simulink model "Golf_Nonlin_Modale"  (R2019a)
settings: Solver=VariableStepAuto  StartTime=0.0  StopTime=300  RelTol=1e-3
values from neighbouring files (symbols this model uses):
  A6 = Acm(iVa:end, iVa:end)    [mainProjetCADV_2a.m]
  alphaTrim = trimVal(2)    [mainProjetCADV_2a.m]
  B6 = Bcm(iVa:end)    [mainProjetCADV_2a.m]
  Cobs = [C6(1,:); C6(3,:); C6(4,:)]    [mainProjetCADV_2a.m]
  Cpf = tf(q(end), minFTBF.num{1})    [mainProjetCADV_2a.m]
  dPHRTrim = trimVal(1)    [mainProjetCADV_2a.m]
  dthrIdle = 0.1    [mainProjetCADV_2a.m]
  H = -inv(C6_pour_h*inv(A6-B6*K_x)*B6)    [mainProjetCADV_2a.m]
  K_i = K_aug(end)    [mainProjetCADV_2a.m]
  K_x = K_aug(1:end-1)    [mainProjetCADV_2a.m]
  km = trim.kmass(choix)    [utGetTrimPoint.m]
  KTS2MS = 1852 / 3600    (= 0.514444444444)    [mainProjetCADV_2a.m]    (also in utAcDynamicsFunction.m)
  L6 = L6t'    [mainProjetCADV_2a.m]
  ms = trim.mStat(choix)    [utGetTrimPoint.m]
  RAD2DEG = 180/pi    (= 57.2957795131)    [mainProjetCADV_2a.m]    (also in utAcDynamicsFunction.m)
  thetaTrim = trimVal(3)    [mainProjetCADV_2a.m]
  uTrim = zeros(TOTAL_CMD, 1)    [mainProjetCADV_2a.m]
  VaTrim = utEas2Tas(Eas_KTS*KTS2MS, hTrimFL*FL2M)    [mainProjetCADV_2a.m]
  xTrim = zeros(TOTAL_SV, 1)    [mainProjetCADV_2a.m]
undefined symbols (not defined in the file or in its folder): aircraftChosen, Eas_KTS, Kd, Ki, Kp
settings Model: Creator=bourdiul  LastModifiedBy=ulyss

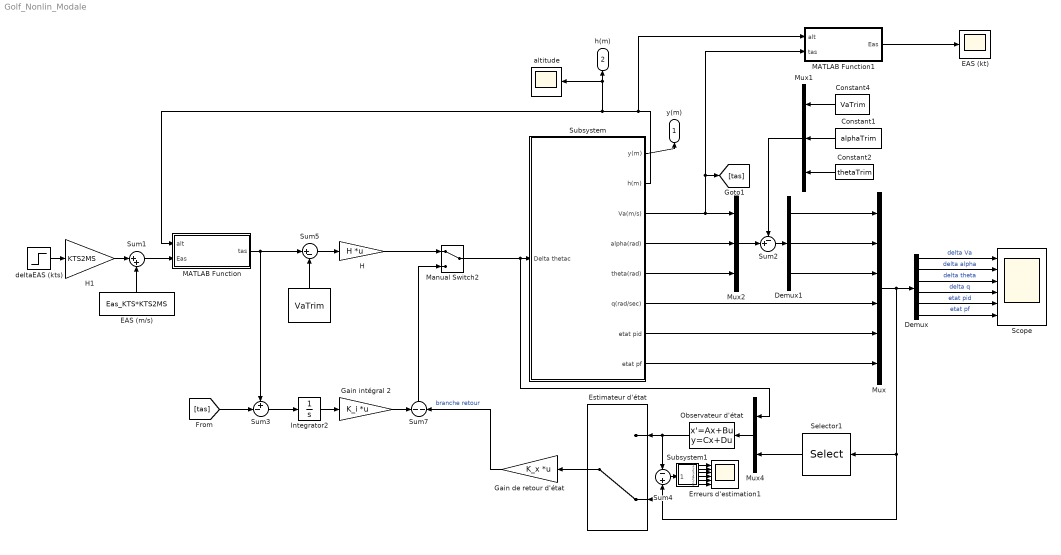
== system Golf_Nonlin_Modale ==
  " " : Constant  Value=VaTrim
  Constant1 : Constant  Value=alphaTrim
  Constant2 : Constant  Value=thetaTrim
  Constant4 : Constant  Value=VaTrim
  Demux : Demux  Outputs=6
  Demux1 : Demux  Outputs=3
  EAS (kt) : Scope
  EAS (m/s) : Constant  Value=Eas_KTS*KTS2MS
  Erreurs d'estimation1 : Scope  NumInputPorts=6
  Estimateur d'état : ManualSwitch  CurrentSetting=0
  Gain de retour d'état : Gain  Gain=K_x  Multiplication=Matrix(K*u) (u vector)
  Gain intégral 2 : Gain  Gain=K_i  Multiplication=Matrix(K*u) (u vector)
  H : Gain  Gain=H  Multiplication=Matrix(K*u) (u vector)
  H1 : Gain  Gain=KTS2MS
  Integrator2 : Integrator
  MATLAB Function : MATLAB Function  TreatAsAtomicUnit=on
  MATLAB Function1 : MATLAB Function  TreatAsAtomicUnit=on
  Manual Switch2 : ManualSwitch
  Mux : Mux  Inputs=6
  Mux1 : Mux  Inputs=3
  Mux2 : Mux  Inputs=3
  Mux4 : Mux  Inputs=2
  Observateur d'état : StateSpace  A=A6-L6*Cobs  B=[B6, L6]  C=eye(6)  D=zeros(6,4)  InitialCondition=0
  Scope : Scope  NumInputPorts=6
  Selector1 : Selector  InputPortWidth=6  IndexOptions=Index vector (dialog)  Indices=[1,3,4]  OutputSizes=1
  Subsystem : Subsystem
  Subsystem1 : Subsystem
  Sum1 : Sum  Inputs=|++
  Sum2 : Sum  Inputs=-+|
  Sum3 : Sum  Inputs=+-|
  Sum4 : Sum  Inputs=-+
  Sum5 : Sum  Inputs=|+-
  Sum7 : Sum  Inputs=-|-
  altitude : Scope
  deltaEAS (kts) : Step  After=2  SampleTime=0
  y(m) : Outport
  h(m) : Outport  Port=2
  wires:
  Demux/6 -> Scope/6  "etat pf"
  H1/1 -> Sum1/1
  Subsystem/1(y(m)) -> y(m)/1
  Subsystem/2(h(m)) -> altitude/1, h(m)/1, MATLAB Function/1(alt), MATLAB Function1/1(alt)
  Sum3/1 -> Integrator2/1
  Subsystem1/6(etat pf) -> Erreurs d'estimation1/6
  Integrator2/1 -> Gain intégral 2/1
  Demux/3 -> Scope/3  "delta theta"
  Sum5/1 -> H/1
  [tas] -> Sum3/2
  Subsystem1/3(delta theta) -> Erreurs d'estimation1/3
  Gain de retour d'état/1 -> Sum7/2  "branche retour"
  Subsystem/4(alpha(rad)) -> Mux2/2
  Demux1/3 -> Mux/3
  Estimateur d'état/1 -> Gain de retour d'état/1
  Subsystem1/5(etat pid) -> Erreurs d'estimation1/5
  Subsystem1/4(delta q) -> Erreurs d'estimation1/4
  Subsystem1/2(delta alpha) -> Erreurs d'estimation1/2
  Sum1/1 -> MATLAB Function/2(Eas)
  Sum4/1 -> Subsystem1/1(In1)
  Subsystem1/1(delta Va) -> Erreurs d'estimation1/1
  Constant2/1 -> Mux1/3
  Selector1/1 -> Mux4/2
  Mux4/1 -> Observateur d'état/1
  H/1 -> Manual Switch2/1
  " "/1 -> Sum5/2
  Observateur d'état/1 -> Sum4/1, Estimateur d'état/1
  Gain intégral 2/1 -> Sum7/1
  Demux/2 -> Scope/2  "delta alpha"
  Constant4/1 -> Mux1/1
  Mux1/1 -> Sum2/1
  Subsystem/5(theta(rad)) -> Mux2/3
  Subsystem/6(q(rad/sec)) -> Mux/4
  Sum7/1 -> Manual Switch2/2
  Subsystem/8("etat pf ") -> Mux/6
  Demux1/2 -> Mux/2
  Demux1/1 -> Mux/1
  Mux/1 -> Sum4/2, Estimateur d'état/2, Selector1/1, Demux/1
  Mux2/1 -> Sum2/2
  Sum2/1 -> Demux1/1
  deltaEAS (kts)/1 -> H1/1
  Constant1/1 -> Mux1/2
  MATLAB Function1/1(Eas) -> EAS (kt)/1
  Manual Switch2/1 -> Mux4/1, Subsystem/1("Delta thetac ")
  Demux/4 -> Scope/4  "delta q"
  Subsystem/7(etat pid) -> Mux/5
  EAS (m/s)/1 -> Sum1/2
  Demux/5 -> Scope/5  "etat pid"
  MATLAB Function/1(tas) -> Sum3/1, Sum5/1
  Demux/1 -> Scope/1  "delta Va"
  Subsystem/3(Va(m/s)) -> Mux2/1, MATLAB Function1/2(tas), [tas]

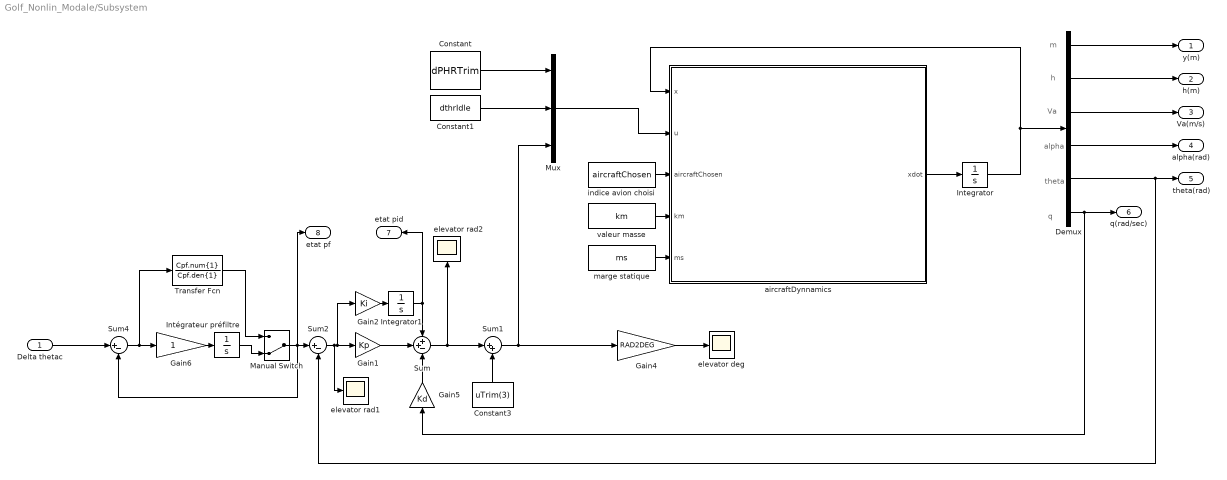
== system Golf_Nonlin_Modale/Subsystem ==
  note: m
  note: h
  note: Va
  note: alpha
  note: theta
  note: q
  "Delta thetac " : Inport
  Constant : Constant  Value=dPHRTrim
  Constant1 : Constant  Value=dthrIdle
  Constant3 : Constant  Value=uTrim(3)
  Demux : Demux  Outputs=6
  Gain1 : Gain  Gain=Kp
  Gain2 : Gain  Gain=Ki
  Gain4 : Gain  Gain=RAD2DEG
  Gain5 : Gain  Gain=Kd
  Gain6 : Gain
  Integrator : Integrator  InitialCondition=xTrim
  Integrator1 : Integrator
  Intégrateur préfiltre : Integrator
  Manual Switch : ManualSwitch  CurrentSetting=0
  Mux : Mux  Inputs=3
  Sum : Sum  Inputs=++-
  Sum1 : Sum  Inputs=|++
  Sum2 : Sum  Inputs=|+-
  Sum4 : Sum  Inputs=|+-
  Transfer Fcn : TransferFcn  Numerator=Cpf.num{1}  Denominator=Cpf.den{1}
  aircraftDynnamics : MATLAB Function  TreatAsAtomicUnit=on
  elevator deg : Scope
  elevator rad1 : Scope
  elevator rad2 : Scope
  indice avion choisi : Constant  Value=aircraftChosen
  marge statique : Constant  Value=ms
  valeur masse : Constant  Value=km
  y(m) : Outport
  h(m) : Outport  Port=2
  Va(m/s) : Outport  Port=3
  alpha(rad) : Outport  Port=4
  theta(rad) : Outport  Port=5
  q(rad/sec) : Outport  Port=6
  etat pid : Outport  Port=7
  "etat pf " : Outport  Port=8
  wires:
  aircraftDynnamics/1(xdot) -> Integrator/1
  "Delta thetac "/1 -> Sum4/1
  Sum1/1 -> Mux/3, Gain4/1
  Sum4/1 -> Gain6/1, Transfer Fcn/1
  Gain2/1 -> Integrator1/1
  Constant/1 -> Mux/1
  Integrator1/1 -> etat pid/1, Sum/1
  Integrator/1 -> aircraftDynnamics/1(x), Demux/1
  Demux/6 -> q(rad/sec)/1, Gain5/1
  Demux/1 -> y(m)/1
  Mux/1 -> aircraftDynnamics/2(u)
  indice avion choisi/1 -> aircraftDynnamics/3(aircraftChosen)
  Gain4/1 -> elevator deg/1
  marge statique/1 -> aircraftDynnamics/5(ms)
  Gain5/1 -> Sum/3
  valeur masse/1 -> aircraftDynnamics/4(km)
  Gain1/1 -> Sum/2
  Demux/4 -> alpha(rad)/1
  Constant3/1 -> Sum1/2
  Gain6/1 -> Intégrateur préfiltre/1
  Demux/2 -> h(m)/1
  Constant1/1 -> Mux/2
  Sum2/1 -> elevator rad1/1, Gain2/1, Gain1/1
  Manual Switch/1 -> Sum4/2, "etat pf "/1, Sum2/1
  Intégrateur préfiltre/1 -> Manual Switch/2
  Transfer Fcn/1 -> Manual Switch/1
  Sum/1 -> Sum1/1, elevator rad2/1
  Demux/5 -> Sum2/2, theta(rad)/1
  Demux/3 -> Va(m/s)/1

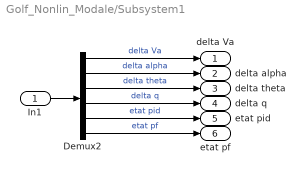
== system Golf_Nonlin_Modale/Subsystem1 ==
  In1 : Inport
  Demux2 : Demux  Outputs=6
  delta Va : Outport
  delta alpha : Outport  Port=2
  delta theta : Outport  Port=3
  delta q : Outport  Port=4
  etat pid : Outport  Port=5
  etat pf : Outport  Port=6
  wires:
  Demux2/3 -> delta theta/1  "delta theta"
  Demux2/1 -> delta Va/1  "delta Va"
  Demux2/6 -> etat pf/1  "etat pf"
  Demux2/5 -> etat pid/1  "etat pid"
  Demux2/2 -> delta alpha/1  "delta alpha"
  In1/1 -> Demux2/1
  Demux2/4 -> delta q/1  "delta q"

== matlab function Golf_Nonlin_Modale/MATLAB Function ==
  data: alt input; Eas input; tas output
function tas = utEas2tas(alt, Eas)
    %tas, Eas (%equivalent vitesse) en m/s
    %alt en m
    %cf. http://www.hochwarth.com/misc/AviationCalculator.html
    tas = sqrt(utRho(0)/utRho(alt))*Eas;
end

== matlab function Golf_Nonlin_Modale/Subsystem/aircraftDynnamics ==
  data: x input; u input; xdot output; aircraftChosen input; km input; ms input
function xdot = aircraftDynamics(x,u, aircraftChosen,km,ms)
    TOTAL_SV = 6;
    xIn = zeros(TOTAL_SV,1);
    xIn = x;
    
	TOTAL_CMD = 3;
    uIn = zeros(TOTAL_CMD,1);
    uIn = u;
    
    xdot = utAcDynamicsFunction(xIn,uIn, aircraftChosen,km,ms);
end %aircraftDynamics

== matlab function Golf_Nonlin_Modale/MATLAB Function1 ==
  data: alt input; tas input; Eas output
function Eas = utTas2Eas(alt, tas)
    %tas, Eas(%equivalent vitesse) en m/s
    %alt en m
    %cf. http://www.hochwarth.com/misc/AviationCalculator.html
    Eas = sqrt(utRho(alt)/utRho(0))*tas/0.5144;
    %sortie en kt
end
